simulink model "hamza_modern_project"  (R2024a)
settings: Solver=FixedStepAuto  StartTime=0.0  StopTime=inf  FixedStep=0.005  RelTol=1e-3
libraries: arduinolib x16, arduinosensorlib x8
settings Model: ExtModeTrigDuration=2  Creator=USER  LastModifiedBy=USER
settings SolverCC: AutoInsertRateTranBlk=on
settings OptimizationCC: EnhancedBackFolding=on  PassReuseOutputArgsAs=Individual arguments  ZeroExternalMemoryAtStartup=off  ZeroInternalMemoryAtStartup=off  MaxStackSize=64  OptimizeBlockOrder=speed  DifferentSizesBufferReuse=on  OptimizationCustomize=off  EfficientTunableParamExpr=on
settings DebuggingCC: ParameterTunabilityLossMsg=error
settings HardwareCC: ProdBitPerInt=16  ProdBitPerPointer=16  ProdBitPerSizeT=16  ProdBitPerPtrDiffT=16  ProdLargestAtomicFloat=None  ProdWordSize=8  ProdHWDeviceType=Atmel->AVR  UseEmbeddedCoderFeatures=off
settings SFSimCC: MATLABDynamicMemAlloc=off
settings RTWCC: Description=Embedded Coder  SystemTargetFile=ert.tlc  HardwareBoard=Arduino Mega 2560  TemplateMakefile=ert_default_tmf  Toolchain=Arduino AVR
settings CodeAppCC: ForceParamTrailComments=on  IgnoreCustomStorageClasses=off  OperatorAnnotations=on  SimulinkDataObjDesc=on  SFDataObjDesc=on  InsertBlockDesc=on
settings ERTTargetCC: SupportContinuousTime=on  SupportNonInlinedSFcns=on  SupportVariableSizeSignals=on  ExtModeTransport=3  ExtModeStaticAlloc=on  ExtModeAutomaticAllocSize=off  ExtModeStaticAllocSize=2048  ExtModeMexFile=ext_xcp  ExtModeIntrfLevel=Level2 - Open

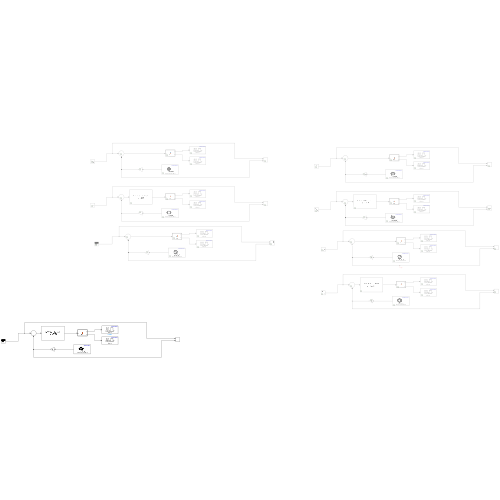
[thumbnail: Simulink's stored preview of the top-level diagram]
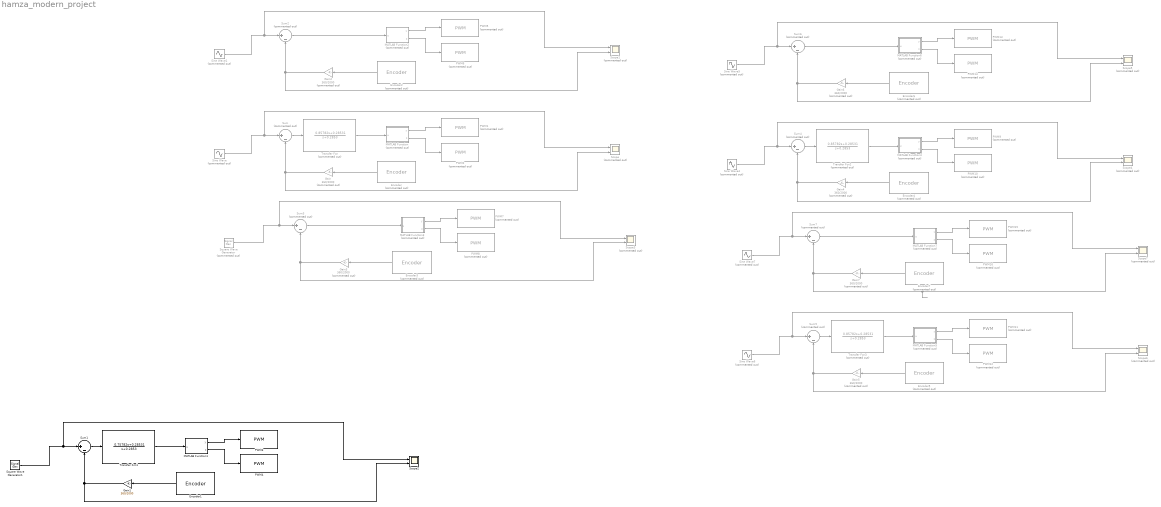
== system hamza_modern_project ==
  Encoder{,2..7} (7 alike) : arduinosensorlib/Encoder  Commented=on  InputA=2  InputB=3  Mode=No reset  SampleTime=-1
  Encoder1 : arduinosensorlib/Encoder  InputA=2  InputB=3  Mode=No reset  SampleTime=-1
  Gain{,2..7} (7 alike) : Gain  Commented=on  Gain=360/2000
  Gain1 : Gain  Gain=360/2000
  MATLAB Function : MATLAB Function  Commented=on  TreatAsAtomicUnit=on
  MATLAB Function1 : MATLAB Function  TreatAsAtomicUnit=on
  MATLAB Function2 : MATLAB Function  Commented=on  TreatAsAtomicUnit=on
  MATLAB Function3 : MATLAB Function  Commented=on  TreatAsAtomicUnit=on
  MATLAB Function4 : MATLAB Function  Commented=on  TreatAsAtomicUnit=on
  MATLAB Function5 : MATLAB Function  Commented=on  TreatAsAtomicUnit=on
  MATLAB Function6 : MATLAB Function  Commented=on  TreatAsAtomicUnit=on
  MATLAB Function7 : MATLAB Function  Commented=on  TreatAsAtomicUnit=on
  PWM{1,5,7,9,11,13,15} (7 alike) : arduinolib/PWM  Commented=on  pinNumber=6  frequencyType=Default  desiredFrequency=490.2  achievableFrequency=490.2
  PWM{2,6,8,10,12,14,16} (7 alike) : arduinolib/PWM  Commented=on  pinNumber=5  frequencyType=Default  desiredFrequency=490.2  achievableFrequency=490.2
  PWM3 : arduinolib/PWM  pinNumber=6  frequencyType=Default  desiredFrequency=490.2  achievableFrequency=490.2
  PWM4 : arduinolib/PWM  pinNumber=5  frequencyType=Default  desiredFrequency=490.2  achievableFrequency=490.2
  Scope{,1,3..7} (7 alike) : Scope  Commented=on  NumInputPorts=2
  Scope2 : Scope  NumInputPorts=2
  Sine Wave : Sin  Commented=on  Amplitude=90  Frequency=100  SampleTime=0
  Sine Wave1 : Sin  Commented=on  Amplitude=90  Frequency=50  SampleTime=0
  Sine Wave4 : Sin  Commented=on  Amplitude=90  Frequency=100  SampleTime=0
  Sine Wave5 : Sin  Commented=on  Amplitude=90  Frequency=50  SampleTime=0
  Sine Wave6 : Sin  Commented=on  Amplitude=90  Frequency=100  SampleTime=0
  Sine Wave7 : Sin  Commented=on  Amplitude=90  Frequency=50  SampleTime=0
  Square Wave Generator : SignalGenerator  Commented=on  WaveForm=square  Amplitude=60  Frequency=50  Units=rad/sec
  Square Wave Generator1 : SignalGenerator  WaveForm=square  Amplitude=60  Frequency=50  Units=rad/sec
  Sum{,2..7} (7 alike) : Sum  Commented=on  Inputs=|+-
  Sum1 : Sum  Inputs=|+-
  Transfer Fcn : TransferFcn  Commented=on  Numerator=[0.85782 0.28531]  Denominator=[1 0.2853]
  Transfer Fcn1 : TransferFcn  Numerator=[0.75782 0.28531]  Denominator=[1 0.2853]
  Transfer Fcn2 : TransferFcn  Commented=on  Numerator=[0.85782 0.28531]  Denominator=[1 0.2853]
  Transfer Fcn3 : TransferFcn  Commented=on  Numerator=[0.85782 0.28531]  Denominator=[1 0.2853]
  wires:
  MATLAB Function/2(z) -> PWM2/1
  MATLAB Function/1(y) -> PWM1/1
  Transfer Fcn/1 -> MATLAB Function/1(u)
  Gain/1 -> Scope/2, Sum/2
  Encoder/1 -> Gain/1
  Sum/1 -> Transfer Fcn/1
  Sine Wave/1 -> Scope/1, Sum/1
  Sine Wave1/1 -> Sum2/1, Scope1/1
  Encoder2/1 -> Gain2/1
  Gain2/1 -> Sum2/2, Scope1/2
  Sum2/1 -> MATLAB Function2/1(u)
  MATLAB Function2/1(y) -> PWM5/1
  MATLAB Function2/2(z) -> PWM6/1
  MATLAB Function3/2(z) -> PWM8/1
  MATLAB Function3/1(y) -> PWM7/1
  Sum3/1 -> MATLAB Function3/1(u)
  Gain3/1 -> Scope3/2, Sum3/2
  Encoder3/1 -> Gain3/1
  Square Wave Generator/1 -> Scope3/1, Sum3/1
  Square Wave Generator1/1 -> Sum1/1, Scope2/1
  Sum1/1 -> Transfer Fcn1/1
  Encoder1/1 -> Gain1/1
  Gain1/1 -> Sum1/2, Scope2/2
  Transfer Fcn1/1 -> MATLAB Function1/1(u)
  MATLAB Function1/1(y) -> PWM3/1
  MATLAB Function1/2(z) -> PWM4/1
  Sine Wave7/1 -> Scope7/1, Sum7/1
  Encoder6/1 -> Gain6/1
  Gain4/1 -> Scope4/2, Sum4/2
  Sine Wave4/1 -> Scope4/1, Sum4/1
  Encoder4/1 -> Gain4/1
  MATLAB Function4/2(z) -> PWM10/1
  MATLAB Function4/1(y) -> PWM9/1
  Transfer Fcn2/1 -> MATLAB Function4/1(u)
  Sine Wave5/1 -> Sum6/1, Scope5/1
  MATLAB Function6/1(y) -> PWM13/1
  MATLAB Function6/2(z) -> PWM14/1
  MATLAB Function7/1(y) -> PWM15/1
  MATLAB Function7/2(z) -> PWM16/1
  Sum4/1 -> Transfer Fcn2/1
  Sine Wave6/1 -> Sum5/1, Scope6/1
  Gain6/1 -> Sum6/2, Scope5/2
  MATLAB Function5/1(y) -> PWM11/1
  MATLAB Function5/2(z) -> PWM12/1
  Gain7/1 -> Scope7/2, Sum7/2
  Transfer Fcn3/1 -> MATLAB Function5/1(u)
  Gain5/1 -> Sum5/2, Scope6/2
  Sum5/1 -> Transfer Fcn3/1
  Encoder7/1 -> Gain7/1
  Sum6/1 -> MATLAB Function6/1(u)
  Sum7/1 -> MATLAB Function7/1(u)
  Encoder5/1 -> Gain5/1

== matlab function hamza_modern_project/MATLAB Function ==
  data: u input; y output; z output
function [y,z] = fcn(u)
    if u == 0
        y = 0;
        z = 0;
    elseif u > 0
        y = 0;
        z = u * 4;
        if (z>255)
            z=255;
        end
    else
        z = 0;
        y = abs(u)* 4;
        if (y>255)
            y=255;
        end
    end
end

== matlab function hamza_modern_project/MATLAB Function2 ==
  data: u input; y output; z output
function [y,z] = fcn(u)
    if u == 0
        y = 0;
        z = 0;
    elseif u > 0
        y = 0;
        z = u * 2;
        if (z>255)
            z=255;
        end
    else
        z = 0;
        y = abs(u)* 2;
        if (y>255)
            y=255;
        end
    end
end

== matlab function hamza_modern_project/MATLAB Function3 ==
  data: u input; y output; z output
function [y,z] = fcn(u)
    if u == 0
        y = 0;
        z = 0;
    elseif u > 0
        y = 0;
        z = u * 2;
        if (z>255)
            z=255;
        end
    else
        z = 0;
        y = abs(u)* 2;
        if (y>255)
            y=255;
        end
    end
end

== matlab function hamza_modern_project/MATLAB Function4 ==
  data: u input; y output; z output
function [y,z] = fcn(u)
    if u == 0
        y = 0;
        z = 0;
    elseif u > 0
        y = 0;
        z = u * 4;
        if (z>255)
            z=255;
        end
    else
        z = 0;
        y = abs(u)* 4;
        if (y>255)
            y=255;
        end
    end
end

== matlab function hamza_modern_project/MATLAB Function5 ==
  data: u input; y output; z output
function [y,z] = fcn(u)
    if u == 0
        y = 0;
        z = 0;
    elseif u > 0
        y = 0;
        z = u * 4;
        if (z>255)
            z=255;
        end
    else
        z = 0;
        y = abs(u)* 4;
        if (y>255)
            y=255;
        end
    end
end

== matlab function hamza_modern_project/MATLAB Function6 ==
  data: u input; y output; z output
function [y,z] = fcn(u)
    if u == 0
        y = 0;
        z = 0;
    elseif u > 0
        y = 0;
        z = u * 2;
        if (z>255)
            z=255;
        end
    else
        z = 0;
        y = abs(u)* 2;
        if (y>255)
            y=255;
        end
    end
end

== matlab function hamza_modern_project/MATLAB Function7 ==
  data: u input; y output; z output
function [y,z] = fcn(u)
    if u == 0
        y = 0;
        z = 0;
    elseif u > 0
        y = 0;
        z = u * 2;
        if (z>255)
            z=255;
        end
    else
        z = 0;
        y = abs(u)* 2;
        if (y>255)
            y=255;
        end
    end
end

== matlab function hamza_modern_project/MATLAB Function1 ==
  data: u input; y output; z output
function [y,z] = fcn(u)
    if u == 0
        y = 0;
        z = 0;
    elseif u > 0
        y = 0;
        z = u * 4;
        if (z>255)
            z=255;
        end
    else
        z = 0;
        y = abs(u)* 4;
        if (y>255)
            y=255;
        end
    end
end
